simulink model "eq6_5"  (R2020a)
settings: Solver=VariableStepAuto  StartTime=0.0  StopTime=10.0  RelTol=1e-3
settings Model: Creator=shrad  LastModifiedBy=shrad

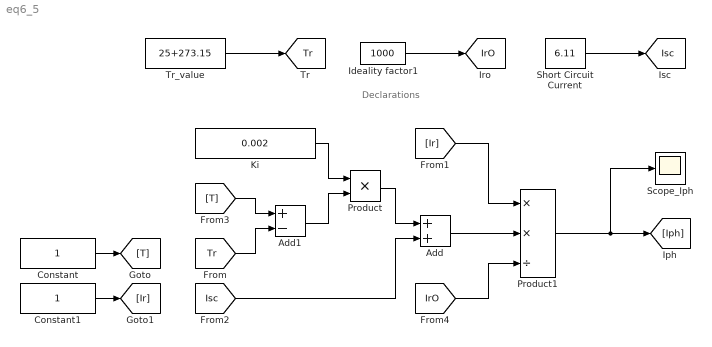
== system eq6_5 ==
  note: Declarations
  Add : Sum
  Add1 : Sum  Inputs=+-
  Constant : Constant
  Constant1 : Constant
  Ideality factor1 : Constant  Value=1000
  Ki : Constant  Value=0.002
  Product : Product
  Product1 : Product  Inputs=**/
  Scope_Iph : Scope
  Short Circuit Current : Constant  Value=6.11
  Tr_value : Constant  Value=25+273.15
  tag scope: IrO=global, Isc=global, Tr=global
  wires:
  Product1/1 -> Scope_Iph/1, [Iph]
  Add1/1 -> Product/2
  [Isc] -> Add/2
  Product/1 -> Add/1
  [Ir] -> Product1/1
  [IrO] -> Product1/3
  [Tr] -> Add1/2
  Add/1 -> Product1/2
  Ki/1 -> Product/1
  [T] -> Add1/1
  Constant/1 -> [T]
  Constant1/1 -> [Ir]
  Short Circuit Current/1 -> [Isc]
  Tr_value/1 -> [Tr]
  Ideality factor1/1 -> [IrO]
